simulink model "simulink_13"  (R2023b)
settings: Solver=FixedStepAuto  StartTime=0.0  StopTime=10.0  FixedStep=0.001  RelTol=1e-3
libraries: simulink x1
(part 3 of 3)

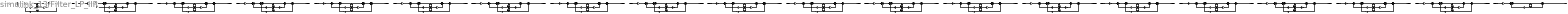
== system simulink_13/Filter_LP_IIR ==
  Input : Inport
  Delay{11..19,21..29,110..120,210..219} (39 alike) : Delay  DelayLength=1  InitialCondition=0
  SumA{21..29,31..39,210..220,310..319} (39 alike) : Sum  Inputs=|+-  RndMeth=Nearest  SaturateOnIntegerOverflow=on  OutDataTypeStr=Inherit: Same as first input
  SumB{21..29,31..39,210..220,310..319} (39 alike) : Sum  Inputs=|++  RndMeth=Nearest  SaturateOnIntegerOverflow=on  OutDataTypeStr=Inherit: Same as first input
  a(2)(1) : Gain  Gain=-1.94511471934265234  ParamDataTypeStr=double  RndMeth=Nearest  SaturateOnIntegerOverflow=on  OutDataTypeStr=Inherit: Same as input
  a(2)(10) : Gain  Gain=-1.72458534142633213  ParamDataTypeStr=double  RndMeth=Nearest  SaturateOnIntegerOverflow=on  OutDataTypeStr=Inherit: Same as input
  a(2)(11) : Gain  Gain=-1.70802795949329655  ParamDataTypeStr=double  RndMeth=Nearest  SaturateOnIntegerOverflow=on  OutDataTypeStr=Inherit: Same as input
  a(2)(12) : Gain  Gain=-1.69318657697153863  ParamDataTypeStr=double  RndMeth=Nearest  SaturateOnIntegerOverflow=on  OutDataTypeStr=Inherit: Same as input
  a(2)(13) : Gain  Gain=-1.6800741629578928  ParamDataTypeStr=double  RndMeth=Nearest  SaturateOnIntegerOverflow=on  OutDataTypeStr=Inherit: Same as input
  a(2)(14) : Gain  Gain=-1.66869977051031126  ParamDataTypeStr=double  RndMeth=Nearest  SaturateOnIntegerOverflow=on  OutDataTypeStr=Inherit: Same as input
  a(2)(15) : Gain  Gain=-1.65906946049562087  ParamDataTypeStr=double  RndMeth=Nearest  SaturateOnIntegerOverflow=on  OutDataTypeStr=Inherit: Same as input
  a(2)(16) : Gain  Gain=-1.6511870851089232  ParamDataTypeStr=double  RndMeth=Nearest  SaturateOnIntegerOverflow=on  OutDataTypeStr=Inherit: Same as input
  a(2)(17) : Gain  Gain=-1.64505493720228069  ParamDataTypeStr=double  RndMeth=Nearest  SaturateOnIntegerOverflow=on  OutDataTypeStr=Inherit: Same as input
  a(2)(18) : Gain  Gain=-1.64067427158636092  ParamDataTypeStr=double  RndMeth=Nearest  SaturateOnIntegerOverflow=on  OutDataTypeStr=Inherit: Same as input
  a(2)(19) : Gain  Gain=-1.63804570396531046  ParamDataTypeStr=double  RndMeth=Nearest  SaturateOnIntegerOverflow=on  OutDataTypeStr=Inherit: Same as input
  a(2)(2) : Gain  Gain=-1.91498797206679394  ParamDataTypeStr=double  RndMeth=Nearest  SaturateOnIntegerOverflow=on  OutDataTypeStr=Inherit: Same as input
  a(2)(20) : Gain  Gain=-0.818584746134231489  ParamDataTypeStr=double  RndMeth=Nearest  SaturateOnIntegerOverflow=on  OutDataTypeStr=Inherit: Same as input
  a(2)(3) : Gain  Gain=-1.88606036875490402  ParamDataTypeStr=double  RndMeth=Nearest  SaturateOnIntegerOverflow=on  OutDataTypeStr=Inherit: Same as input
  a(2)(4) : Gain  Gain=-1.85844504972081848  ParamDataTypeStr=double  RndMeth=Nearest  SaturateOnIntegerOverflow=on  OutDataTypeStr=Inherit: Same as input
  a(2)(5) : Gain  Gain=-1.8322368670218232  ParamDataTypeStr=double  RndMeth=Nearest  SaturateOnIntegerOverflow=on  OutDataTypeStr=Inherit: Same as input
  a(2)(6) : Gain  Gain=-1.80751433005880968  ParamDataTypeStr=double  RndMeth=Nearest  SaturateOnIntegerOverflow=on  OutDataTypeStr=Inherit: Same as input
  a(2)(7) : Gain  Gain=-1.78434154259198308  ParamDataTypeStr=double  RndMeth=Nearest  SaturateOnIntegerOverflow=on  OutDataTypeStr=Inherit: Same as input
  a(2)(8) : Gain  Gain=-1.76277007981037737  ParamDataTypeStr=double  RndMeth=Nearest  SaturateOnIntegerOverflow=on  OutDataTypeStr=Inherit: Same as input
  a(2)(9) : Gain  Gain=-1.74284076803979437  ParamDataTypeStr=double  RndMeth=Nearest  SaturateOnIntegerOverflow=on  OutDataTypeStr=Inherit: Same as input
  a(3)(1) : Gain  Gain=0.984216738021379101  ParamDataTypeStr=double  RndMeth=Nearest  SaturateOnIntegerOverflow=on  OutDataTypeStr=Inherit: Same as input
  a(3)(10) : Gain  Gain=0.75925412860012953  ParamDataTypeStr=double  RndMeth=Nearest  SaturateOnIntegerOverflow=on  OutDataTypeStr=Inherit: Same as input
  a(3)(11) : Gain  Gain=0.742363898917201115  ParamDataTypeStr=double  RndMeth=Nearest  SaturateOnIntegerOverflow=on  OutDataTypeStr=Inherit: Same as input
  a(3)(12) : Gain  Gain=0.727224164832518616  ParamDataTypeStr=double  RndMeth=Nearest  SaturateOnIntegerOverflow=on  OutDataTypeStr=Inherit: Same as input
  a(3)(13) : Gain  Gain=0.713848156156518643  ParamDataTypeStr=double  RndMeth=Nearest  SaturateOnIntegerOverflow=on  OutDataTypeStr=Inherit: Same as input
  a(3)(14) : Gain  Gain=0.702245107937880753  ParamDataTypeStr=double  RndMeth=Nearest  SaturateOnIntegerOverflow=on  OutDataTypeStr=Inherit: Same as input
  a(3)(15) : Gain  Gain=0.692421202883097386  ParamDataTypeStr=double  RndMeth=Nearest  SaturateOnIntegerOverflow=on  OutDataTypeStr=Inherit: Same as input
  a(3)(16) : Gain  Gain=0.684380370626715751  ParamDataTypeStr=double  RndMeth=Nearest  SaturateOnIntegerOverflow=on  OutDataTypeStr=Inherit: Same as input
  a(3)(17) : Gain  Gain=0.67812495011326912  ParamDataTypeStr=double  RndMeth=Nearest  SaturateOnIntegerOverflow=on  OutDataTypeStr=Inherit: Same as input
  a(3)(18) : Gain  Gain=0.6736562213784828  ParamDataTypeStr=double  RndMeth=Nearest  SaturateOnIntegerOverflow=on  OutDataTypeStr=Inherit: Same as input
  a(3)(19) : Gain  Gain=0.670974812503806195  ParamDataTypeStr=double  RndMeth=Nearest  SaturateOnIntegerOverflow=on  OutDataTypeStr=Inherit: Same as input
  a(3)(2) : Gain  Gain=0.953484362386948781  ParamDataTypeStr=double  RndMeth=Nearest  SaturateOnIntegerOverflow=on  OutDataTypeStr=Inherit: Same as input
  a(3)(3) : Gain  Gain=0.92397523672381443  ParamDataTypeStr=double  RndMeth=Nearest  SaturateOnIntegerOverflow=on  OutDataTypeStr=Inherit: Same as input
  a(3)(4) : Gain  Gain=0.895804775769331041  ParamDataTypeStr=double  RndMeth=Nearest  SaturateOnIntegerOverflow=on  OutDataTypeStr=Inherit: Same as input
  a(3)(5) : Gain  Gain=0.869069738361335387  ParamDataTypeStr=double  RndMeth=Nearest  SaturateOnIntegerOverflow=on  OutDataTypeStr=Inherit: Same as input
  a(3)(6) : Gain  Gain=0.843850212150078494  ParamDataTypeStr=double  RndMeth=Nearest  SaturateOnIntegerOverflow=on  OutDataTypeStr=Inherit: Same as input
  a(3)(7) : Gain  Gain=0.820211589553140663  ParamDataTypeStr=double  RndMeth=Nearest  SaturateOnIntegerOverflow=on  OutDataTypeStr=Inherit: Same as input
  a(3)(8) : Gain  Gain=0.798206482559074892  ParamDataTypeStr=double  RndMeth=Nearest  SaturateOnIntegerOverflow=on  OutDataTypeStr=Inherit: Same as input
  a(3)(9) : Gain  Gain=0.777876538212244339  ParamDataTypeStr=double  RndMeth=Nearest  SaturateOnIntegerOverflow=on  OutDataTypeStr=Inherit: Same as input
  b(2)(1) : Gain  Gain=2  ParamDataTypeStr=double  RndMeth=Nearest  SaturateOnIntegerOverflow=on  OutDataTypeStr=Inherit: Same as input
  b(2)(10) : Gain  Gain=2  ParamDataTypeStr=double  RndMeth=Nearest  SaturateOnIntegerOverflow=on  OutDataTypeStr=Inherit: Same as input
  b(2)(11) : Gain  Gain=2  ParamDataTypeStr=double  RndMeth=Nearest  SaturateOnIntegerOverflow=on  OutDataTypeStr=Inherit: Same as input
  b(2)(12) : Gain  Gain=2  ParamDataTypeStr=double  RndMeth=Nearest  SaturateOnIntegerOverflow=on  OutDataTypeStr=Inherit: Same as input
  b(2)(13) : Gain  Gain=2  ParamDataTypeStr=double  RndMeth=Nearest  SaturateOnIntegerOverflow=on  OutDataTypeStr=Inherit: Same as input
  b(2)(14) : Gain  Gain=2  ParamDataTypeStr=double  RndMeth=Nearest  SaturateOnIntegerOverflow=on  OutDataTypeStr=Inherit: Same as input
  b(2)(15) : Gain  Gain=2  ParamDataTypeStr=double  RndMeth=Nearest  SaturateOnIntegerOverflow=on  OutDataTypeStr=Inherit: Same as input
  b(2)(16) : Gain  Gain=2  ParamDataTypeStr=double  RndMeth=Nearest  SaturateOnIntegerOverflow=on  OutDataTypeStr=Inherit: Same as input
  b(2)(17) : Gain  Gain=2  ParamDataTypeStr=double  RndMeth=Nearest  SaturateOnIntegerOverflow=on  OutDataTypeStr=Inherit: Same as input
  b(2)(18) : Gain  Gain=2  ParamDataTypeStr=double  RndMeth=Nearest  SaturateOnIntegerOverflow=on  OutDataTypeStr=Inherit: Same as input
  b(2)(19) : Gain  Gain=2  ParamDataTypeStr=double  RndMeth=Nearest  SaturateOnIntegerOverflow=on  OutDataTypeStr=Inherit: Same as input
  b(2)(2) : Gain  Gain=2  ParamDataTypeStr=double  RndMeth=Nearest  SaturateOnIntegerOverflow=on  OutDataTypeStr=Inherit: Same as input
  b(2)(3) : Gain  Gain=2  ParamDataTypeStr=double  RndMeth=Nearest  SaturateOnIntegerOverflow=on  OutDataTypeStr=Inherit: Same as input
  b(2)(4) : Gain  Gain=2  ParamDataTypeStr=double  RndMeth=Nearest  SaturateOnIntegerOverflow=on  OutDataTypeStr=Inherit: Same as input
  b(2)(5) : Gain  Gain=2  ParamDataTypeStr=double  RndMeth=Nearest  SaturateOnIntegerOverflow=on  OutDataTypeStr=Inherit: Same as input
  b(2)(6) : Gain  Gain=2  ParamDataTypeStr=double  RndMeth=Nearest  SaturateOnIntegerOverflow=on  OutDataTypeStr=Inherit: Same as input
  b(2)(7) : Gain  Gain=2  ParamDataTypeStr=double  RndMeth=Nearest  SaturateOnIntegerOverflow=on  OutDataTypeStr=Inherit: Same as input
  b(2)(8) : Gain  Gain=2  ParamDataTypeStr=double  RndMeth=Nearest  SaturateOnIntegerOverflow=on  OutDataTypeStr=Inherit: Same as input
  b(2)(9) : Gain  Gain=2  ParamDataTypeStr=double  RndMeth=Nearest  SaturateOnIntegerOverflow=on  OutDataTypeStr=Inherit: Same as input
  s(1) : Gain  Gain=0.00977550466968172584  ParamDataTypeStr=double  RndMeth=Nearest  SaturateOnIntegerOverflow=on  OutDataTypeStr=Inherit: Same as input
  s(10) : Gain  Gain=0.00866719679344934817  ParamDataTypeStr=double  RndMeth=Nearest  SaturateOnIntegerOverflow=on  OutDataTypeStr=Inherit: Same as input
  s(11) : Gain  Gain=0.00858398485597617299  ParamDataTypeStr=double  RndMeth=Nearest  SaturateOnIntegerOverflow=on  OutDataTypeStr=Inherit: Same as input
  s(12) : Gain  Gain=0.00850939696524497316  ParamDataTypeStr=double  RndMeth=Nearest  SaturateOnIntegerOverflow=on  OutDataTypeStr=Inherit: Same as input
  s(13) : Gain  Gain=0.00844349829965649126  ParamDataTypeStr=double  RndMeth=Nearest  SaturateOnIntegerOverflow=on  OutDataTypeStr=Inherit: Same as input
  s(14) : Gain  Gain=0.0083863343568923842  ParamDataTypeStr=double  RndMeth=Nearest  SaturateOnIntegerOverflow=on  OutDataTypeStr=Inherit: Same as input
  s(15) : Gain  Gain=0.00833793559686916812  ParamDataTypeStr=double  RndMeth=Nearest  SaturateOnIntegerOverflow=on  OutDataTypeStr=Inherit: Same as input
  s(16) : Gain  Gain=0.00829832137944815779  ParamDataTypeStr=double  RndMeth=Nearest  SaturateOnIntegerOverflow=on  OutDataTypeStr=Inherit: Same as input
  s(17) : Gain  Gain=0.0082675032277471517  ParamDataTypeStr=double  RndMeth=Nearest  SaturateOnIntegerOverflow=on  OutDataTypeStr=Inherit: Same as input
  s(18) : Gain  Gain=0.00824548744803046268  ParamDataTypeStr=double  RndMeth=Nearest  SaturateOnIntegerOverflow=on  OutDataTypeStr=Inherit: Same as input
  s(19) : Gain  Gain=0.00823227713462394185  ParamDataTypeStr=double  RndMeth=Nearest  SaturateOnIntegerOverflow=on  OutDataTypeStr=Inherit: Same as input
  s(2) : Gain  Gain=0.00962409758003870443  ParamDataTypeStr=double  RndMeth=Nearest  SaturateOnIntegerOverflow=on  OutDataTypeStr=Inherit: Same as input
  s(20) : Gain  Gain=0.0907076269328842  ParamDataTypeStr=double  RndMeth=Nearest  SaturateOnIntegerOverflow=on  OutDataTypeStr=Inherit: Same as input
  s(3) : Gain  Gain=0.00947871699222759163  ParamDataTypeStr=double  RndMeth=Nearest  SaturateOnIntegerOverflow=on  OutDataTypeStr=Inherit: Same as input
  s(4) : Gain  Gain=0.00933993151212815335  ParamDataTypeStr=double  RndMeth=Nearest  SaturateOnIntegerOverflow=on  OutDataTypeStr=Inherit: Same as input
  s(5) : Gain  Gain=0.00920821783487806196  ParamDataTypeStr=double  RndMeth=Nearest  SaturateOnIntegerOverflow=on  OutDataTypeStr=Inherit: Same as input
  s(6) : Gain  Gain=0.00908397052281721337  ParamDataTypeStr=double  RndMeth=Nearest  SaturateOnIntegerOverflow=on  OutDataTypeStr=Inherit: Same as input
  s(7) : Gain  Gain=0.00896751174028943485  ParamDataTypeStr=double  RndMeth=Nearest  SaturateOnIntegerOverflow=on  OutDataTypeStr=Inherit: Same as input
  s(8) : Gain  Gain=0.00885910068717442149  ParamDataTypeStr=double  RndMeth=Nearest  SaturateOnIntegerOverflow=on  OutDataTypeStr=Inherit: Same as input
  s(9) : Gain  Gain=0.00875894254311250509  ParamDataTypeStr=double  RndMeth=Nearest  SaturateOnIntegerOverflow=on  OutDataTypeStr=Inherit: Same as input
  Output : Outport
  wires:
  Input/1 -> s(1)/1
  s(1)/1 -> SumA21/1
  SumA21/1 -> SumA31/1
  SumA31/1 -> SumB21/1, Delay11/1
  SumB21/1 -> SumB31/1
  SumB31/1 -> [Sect1]
  a(2)(1)/1 -> SumA21/2
  Delay11/1 -> a(2)(1)/1, b(2)(1)/1, Delay21/1
  b(2)(1)/1 -> SumB21/2
  a(3)(1)/1 -> SumA31/2
  Delay21/1 -> a(3)(1)/1, SumB31/2
  [Sect1] -> s(2)/1
  s(2)/1 -> SumA22/1
  SumA22/1 -> SumA32/1
  SumA32/1 -> SumB22/1, Delay12/1
  SumB22/1 -> SumB32/1
  SumB32/1 -> [Sect2]
  a(2)(2)/1 -> SumA22/2
  Delay12/1 -> a(2)(2)/1, b(2)(2)/1, Delay22/1
  b(2)(2)/1 -> SumB22/2
  a(3)(2)/1 -> SumA32/2
  Delay22/1 -> a(3)(2)/1, SumB32/2
  [Sect2] -> s(3)/1
  s(3)/1 -> SumA23/1
  SumA23/1 -> SumA33/1
  SumA33/1 -> SumB23/1, Delay13/1
  SumB23/1 -> SumB33/1
  SumB33/1 -> [Sect3]
  a(2)(3)/1 -> SumA23/2
  Delay13/1 -> a(2)(3)/1, b(2)(3)/1, Delay23/1
  b(2)(3)/1 -> SumB23/2
  a(3)(3)/1 -> SumA33/2
  Delay23/1 -> a(3)(3)/1, SumB33/2
  [Sect3] -> s(4)/1
  s(4)/1 -> SumA24/1
  SumA24/1 -> SumA34/1
  SumA34/1 -> SumB24/1, Delay14/1
  SumB24/1 -> SumB34/1
  SumB34/1 -> [Sect4]
  a(2)(4)/1 -> SumA24/2
  Delay14/1 -> a(2)(4)/1, b(2)(4)/1, Delay24/1
  b(2)(4)/1 -> SumB24/2
  a(3)(4)/1 -> SumA34/2
  Delay24/1 -> a(3)(4)/1, SumB34/2
  [Sect4] -> s(5)/1
  s(5)/1 -> SumA25/1
  SumA25/1 -> SumA35/1
  SumA35/1 -> SumB25/1, Delay15/1
  SumB25/1 -> SumB35/1
  SumB35/1 -> [Sect5]
  a(2)(5)/1 -> SumA25/2
  Delay15/1 -> a(2)(5)/1, b(2)(5)/1, Delay25/1
  b(2)(5)/1 -> SumB25/2
  a(3)(5)/1 -> SumA35/2
  Delay25/1 -> a(3)(5)/1, SumB35/2
  [Sect5] -> s(6)/1
  s(6)/1 -> SumA26/1
  SumA26/1 -> SumA36/1
  SumA36/1 -> SumB26/1, Delay16/1
  SumB26/1 -> SumB36/1
  SumB36/1 -> [Sect6]
  a(2)(6)/1 -> SumA26/2
  Delay16/1 -> a(2)(6)/1, b(2)(6)/1, Delay26/1
  b(2)(6)/1 -> SumB26/2
  a(3)(6)/1 -> SumA36/2
  Delay26/1 -> a(3)(6)/1, SumB36/2
  [Sect6] -> s(7)/1
  s(7)/1 -> SumA27/1
  SumA27/1 -> SumA37/1
  SumA37/1 -> SumB27/1, Delay17/1
  SumB27/1 -> SumB37/1
  SumB37/1 -> [Sect7]
  a(2)(7)/1 -> SumA27/2
  Delay17/1 -> a(2)(7)/1, b(2)(7)/1, Delay27/1
  b(2)(7)/1 -> SumB27/2
  a(3)(7)/1 -> SumA37/2
  Delay27/1 -> a(3)(7)/1, SumB37/2
  [Sect7] -> s(8)/1
  s(8)/1 -> SumA28/1
  SumA28/1 -> SumA38/1
  SumA38/1 -> SumB28/1, Delay18/1
  SumB28/1 -> SumB38/1
  SumB38/1 -> [Sect8]
  a(2)(8)/1 -> SumA28/2
  Delay18/1 -> a(2)(8)/1, b(2)(8)/1, Delay28/1
  b(2)(8)/1 -> SumB28/2
  a(3)(8)/1 -> SumA38/2
  Delay28/1 -> a(3)(8)/1, SumB38/2
  [Sect8] -> s(9)/1
  s(9)/1 -> SumA29/1
  SumA29/1 -> SumA39/1
  SumA39/1 -> SumB29/1, Delay19/1
  SumB29/1 -> SumB39/1
  SumB39/1 -> [Sect9]
  a(2)(9)/1 -> SumA29/2
  Delay19/1 -> a(2)(9)/1, b(2)(9)/1, Delay29/1
  b(2)(9)/1 -> SumB29/2
  a(3)(9)/1 -> SumA39/2
  Delay29/1 -> a(3)(9)/1, SumB39/2
  [Sect9] -> s(10)/1
  s(10)/1 -> SumA210/1
  SumA210/1 -> SumA310/1
  SumA310/1 -> SumB210/1, Delay110/1
  SumB210/1 -> SumB310/1
  SumB310/1 -> [Sect10]
  a(2)(10)/1 -> SumA210/2
  Delay110/1 -> a(2)(10)/1, b(2)(10)/1, Delay210/1
  b(2)(10)/1 -> SumB210/2
  a(3)(10)/1 -> SumA310/2
  Delay210/1 -> a(3)(10)/1, SumB310/2
  [Sect10] -> s(11)/1
  s(11)/1 -> SumA211/1
  SumA211/1 -> SumA311/1
  SumA311/1 -> SumB211/1, Delay111/1
  SumB211/1 -> SumB311/1
  SumB311/1 -> [Sect11]
  a(2)(11)/1 -> SumA211/2
  Delay111/1 -> a(2)(11)/1, b(2)(11)/1, Delay211/1
  b(2)(11)/1 -> SumB211/2
  a(3)(11)/1 -> SumA311/2
  Delay211/1 -> a(3)(11)/1, SumB311/2
  [Sect11] -> s(12)/1
  s(12)/1 -> SumA212/1
  SumA212/1 -> SumA312/1
  SumA312/1 -> SumB212/1, Delay112/1
  SumB212/1 -> SumB312/1
  SumB312/1 -> [Sect12]
  a(2)(12)/1 -> SumA212/2
  Delay112/1 -> a(2)(12)/1, b(2)(12)/1, Delay212/1
  b(2)(12)/1 -> SumB212/2
  a(3)(12)/1 -> SumA312/2
  Delay212/1 -> a(3)(12)/1, SumB312/2
  [Sect12] -> s(13)/1
  s(13)/1 -> SumA213/1
  SumA213/1 -> SumA313/1
  SumA313/1 -> SumB213/1, Delay113/1
  SumB213/1 -> SumB313/1
  SumB313/1 -> [Sect13]
  a(2)(13)/1 -> SumA213/2
  Delay113/1 -> a(2)(13)/1, b(2)(13)/1, Delay213/1
  b(2)(13)/1 -> SumB213/2
  a(3)(13)/1 -> SumA313/2
  Delay213/1 -> a(3)(13)/1, SumB313/2
  [Sect13] -> s(14)/1
  s(14)/1 -> SumA214/1
  SumA214/1 -> SumA314/1
  SumA314/1 -> SumB214/1, Delay114/1
  SumB214/1 -> SumB314/1
  SumB314/1 -> [Sect14]
  a(2)(14)/1 -> SumA214/2
  Delay114/1 -> a(2)(14)/1, b(2)(14)/1, Delay214/1
  b(2)(14)/1 -> SumB214/2
  a(3)(14)/1 -> SumA314/2
  Delay214/1 -> a(3)(14)/1, SumB314/2
  [Sect14] -> s(15)/1
  s(15)/1 -> SumA215/1
  SumA215/1 -> SumA315/1
  SumA315/1 -> SumB215/1, Delay115/1
  SumB215/1 -> SumB315/1
  SumB315/1 -> [Sect15]
  a(2)(15)/1 -> SumA215/2
  Delay115/1 -> a(2)(15)/1, b(2)(15)/1, Delay215/1
  b(2)(15)/1 -> SumB215/2
  a(3)(15)/1 -> SumA315/2
  Delay215/1 -> a(3)(15)/1, SumB315/2
  [Sect15] -> s(16)/1
  s(16)/1 -> SumA216/1
  SumA216/1 -> SumA316/1
  SumA316/1 -> SumB216/1, Delay116/1
  SumB216/1 -> SumB316/1
  SumB316/1 -> [Sect16]
  a(2)(16)/1 -> SumA216/2
  Delay116/1 -> a(2)(16)/1, b(2)(16)/1, Delay216/1
  b(2)(16)/1 -> SumB216/2
  a(3)(16)/1 -> SumA316/2
  Delay216/1 -> a(3)(16)/1, SumB316/2
  [Sect16] -> s(17)/1
  s(17)/1 -> SumA217/1
  SumA217/1 -> SumA317/1
  SumA317/1 -> SumB217/1, Delay117/1
  SumB217/1 -> SumB317/1
  SumB317/1 -> [Sect17]
  a(2)(17)/1 -> SumA217/2
  Delay117/1 -> a(2)(17)/1, b(2)(17)/1, Delay217/1
  b(2)(17)/1 -> SumB217/2
  a(3)(17)/1 -> SumA317/2
  Delay217/1 -> a(3)(17)/1, SumB317/2
  [Sect17] -> s(18)/1
  s(18)/1 -> SumA218/1
  SumA218/1 -> SumA318/1
  SumA318/1 -> SumB218/1, Delay118/1
  SumB218/1 -> SumB318/1
  SumB318/1 -> [Sect18]
  a(2)(18)/1 -> SumA218/2
  Delay118/1 -> a(2)(18)/1, b(2)(18)/1, Delay218/1
  b(2)(18)/1 -> SumB218/2
  a(3)(18)/1 -> SumA318/2
  Delay218/1 -> a(3)(18)/1, SumB318/2
  [Sect18] -> s(19)/1
  s(19)/1 -> SumA219/1
  SumA219/1 -> SumA319/1
  SumA319/1 -> SumB219/1, Delay119/1
  SumB219/1 -> SumB319/1
  SumB319/1 -> [Sect19]
  a(2)(19)/1 -> SumA219/2
  Delay119/1 -> a(2)(19)/1, b(2)(19)/1, Delay219/1
  b(2)(19)/1 -> SumB219/2
  a(3)(19)/1 -> SumA319/2
  Delay219/1 -> a(3)(19)/1, SumB319/2
  [Sect19] -> s(20)/1
  s(20)/1 -> SumA220/1
  SumA220/1 -> SumB220/1, Delay120/1
  SumB220/1 -> Output/1
  a(2)(20)/1 -> SumA220/2
  Delay120/1 -> a(2)(20)/1, SumB220/2
